simulink model "Moteurs_PLA"  (R2020b)
settings: Solver=FixedStepAuto  StartTime=0.0  StopTime=tsim+0.2  FixedStep=0.001  RelTol=1e-3
values from neighbouring files (symbols this model uses):
  X = C.Data(:,1,:)    [Initiliastion_PLA.m]
  x0 = -0.3929    [Simulation_PLA.m]
  x1 = -0.3929    [Simulation_PLA.m]
  xraten = a    (= 0)    [Simulation_PLA.m]
  xratep = 0    [Simulation_PLA.m]
  Y = C.Data(:,2,:)    [Initiliastion_PLA.m]
  y0 = -0.006639    [Simulation_PLA.m]
  y1 = -0.006639    [Simulation_PLA.m]
  yraten = b    (= 0)    [Simulation_PLA.m]
  yratep = 0    [Simulation_PLA.m]
  Z = C.Data(:,3,:)    [Initiliastion_PLA.m]
  z0 = 0.25    [Simulation_PLA.m]
  z1 = 0.25    [Simulation_PLA.m]
  zraten = c    (= 0)    [Simulation_PLA.m]
  zratep = 0    [Simulation_PLA.m]
undefined symbols (not defined in the file or in its folder): Levenberg, Marquardt, smiData
libraries: sm_lib x404, nesl_utility x24, robotcorelib x1, robotmaniplib x1
(part 1 of 7)
settings Model: Creator=alessandrini  LastModifiedBy=alessandrini
settings ExplorerConfigSet: InternalSimMechanicsExplorerSettings="<ExplorerConfiguration><canonicalview>default</canonicalview><AnimationSetting><BasePlaybackSpeed>1.0</BasePlaybackSpeed><PlaybackSpeedFactor>1.0</PlaybackSpeedFactor></AnimationSetting><TilePanel><TileInfo><Tiles Columns=\"1\" Count=\"1\" Rows=\"1\"><Column Weight=\"1\"/><Row Weight=\"1\"/><Tile Height=\"1\" Width=\"1\" X=\"0\" Y=\"0\"/></Tiles></TileInfo><SceneInfo><SceneViewer><BGColor><R>1</R><G>1</G><B>1</B></BGColor><Camera><DoPerspective>off</DoPerspective><Position><X>0.443375350255403866</X><Y>-0.57400040031573929</Y><Z>0.816945670282958059</Z></Position><Center><X>-0.133974918934221976</X><Y>0.00334986887388660781</Y><Z>0.239595401093332216</Z></Center><Up><X>-0.408248290463863073</X><Y>0.408248290463863073</Y><Z>0.816496580927726145</Z></Up><ViewLimDist>1</ViewLimDist><YLim>0.387829513549804716</YLim><XLim>0.326078018188476593</XLim></Camera></SceneViewer></SceneInfo></TilePanel><MechEditorPanel><Cameras/><GfxPanelCameraMap/><VideoCreator><PlaybackSpeedRatio>1.0</PlaybackSpeedRatio><FrameRate>30</FrameRate><VideoFormat>Motion JPEG AVI</VideoFormat><FrameSize>auto</FrameSize></VideoCreator></MechEditorPanel></ExplorerConfiguration>"

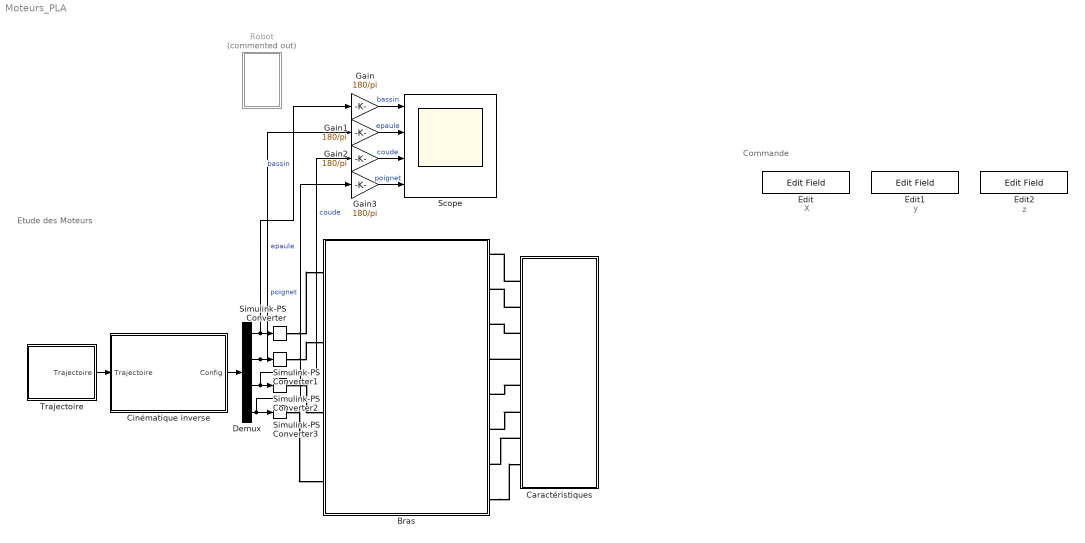
== system Moteurs_PLA ==
  note: Commande
  note: z
  note: y
  note: X
  note: Etude des Moteurs
  Bras : Subsystem
  Caractéristiques : Subsystem
  Cinématique inverse : Subsystem
  Demux : Demux
  Edit : EditField  LabelPosition=Hide  ShowInitialText=on  Alignment=Center
  Edit1 : EditField  LabelPosition=Hide  ShowInitialText=on  Alignment=Center
  Edit2 : EditField  LabelPosition=Hide  ShowInitialText=on  Alignment=Center
  Gain{,1..3} (4 alike) : Gain  Gain=180/pi
  Robot : Subsystem  Commented=on
  Scope : Scope  NumInputPorts=4
  Simulink-PS Converter{,1..3} (4 alike) : nesl_utility/Simulink-PS Converter  PhysicalDomain=network_engine_domain  SubClassName=ps_input  LeftPortType=input  RightPortType=output  PseudoPeriodic=off  Frequencies=[]  NoiseDistribution=none  NoiseParameters=[]  Unit=1  AffineConversion=off  FilteringAndDerivatives=filter  SimscapeFilterOrder=2  InputFilterTimeConstant=0.001  UdotUserProvided=0
  Trajectoire : Subsystem
  wires:
  Trajectoire/1(Trajectoire) -> Cinématique inverse/1(Trajectoire)
  Demux/4 -> Gain3/1, Simulink-PS Converter3/1  "poignet"
  Cinématique inverse/1(Config) -> Demux/1
  Gain/1 -> Scope/1  "bassin"
  Gain2/1 -> Scope/3  "coude"
  Demux/2 -> Gain1/1, Simulink-PS Converter1/1  "epaule"
  Gain1/1 -> Scope/2  "epaule"
  Demux/1 -> Gain/1, Simulink-PS Converter/1  "bassin"
  Demux/3 -> Gain2/1, Simulink-PS Converter2/1  "coude"
  Gain3/1 -> Scope/4  "poignet"
  connections:
  Caractéristiques/LConn1 -- Bras/RConn1
  Caractéristiques/LConn3 -- Bras/RConn3
  Caractéristiques/LConn5 -- Bras/RConn5
  Simulink-PS Converter1/RConn1 -- Bras/LConn2
  Caractéristiques/LConn4 -- Bras/RConn4
  Caractéristiques/LConn2 -- Bras/RConn2
  Caractéristiques/LConn6 -- Bras/RConn6
  Simulink-PS Converter/RConn1 -- Bras/LConn1
  Caractéristiques/LConn7 -- Bras/RConn7
  Simulink-PS Converter2/RConn1 -- Bras/LConn3
  Simulink-PS Converter3/RConn1 -- Bras/LConn4
  Bras/RConn8 -- Caractéristiques/LConn8

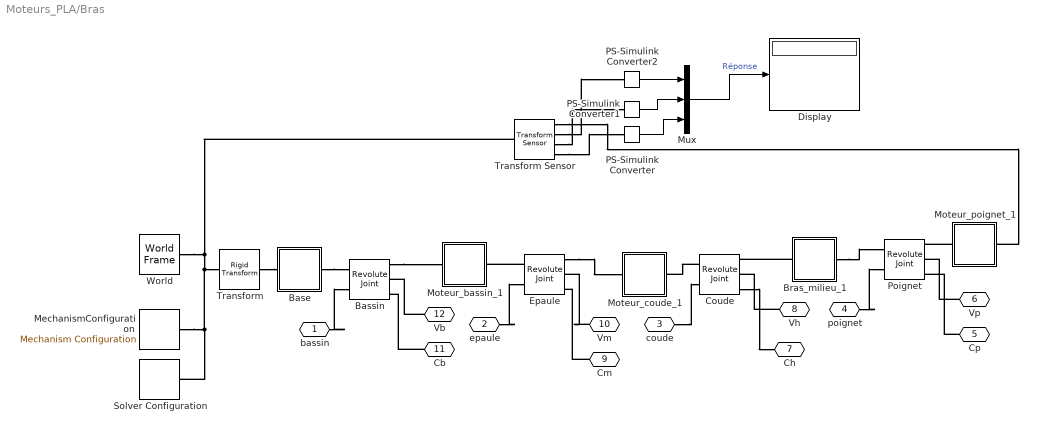
== system Moteurs_PLA/Bras ==
  Base : Subsystem
  Bassin : sm_lib/Joints/Revolute Joint  JointMode=Normal  SenseConstraintForce=off  SenseConstraintForceX=off  SenseConstraintForceY=off  SenseConstraintForceZ=off  SenseConstraintTorque=off  SenseConstraintTorqueX=off  SenseConstraintTorqueY=off  SenseConstraintTorqueZ=off  SenseTotalForce=off  SenseTotalForceX=off  SenseTotalForceY=off  SenseTotalForceZ=off  SenseTotalTorque=off  SenseTotalTorqueX=off  SenseTotalTorqueY=off  SenseTotalTorqueZ=off  CompositeWrenchDir=FollowerOnBase  CompositeWrenchFrame=BaseFrame  EquilibriumPosition=0  EquilibriumPositionUnits=deg  SpringStiffness=0  SpringStiffnessUnits=N*m/deg  DampingCoefficient=0  DampingCoefficientUnits=N*m/(deg/s)  TorqueActuationMode=ComputedTorque  MotionActuationMode=InputMotion  SensePosition=off  SenseVelocity=on  SenseAcceleration=off  SenseTorqueForce=on  SenseLowerLimitTorqueForce=off  SenseUpperLimitTorqueForce=off  LowerLimitSpecify=off  LowerLimitBound=-180  LowerLimitBoundUnits=deg  LowerLimitStiffness=1e4  LowerLimitStiffnessUnits=N*m/deg  LowerLimitDamping=10  LowerLimitDampingUnits=N*m/(deg/s)  LowerLimitTransitionRegionWidth=0.1  LowerLimitTransitionRegionWidthUnits=deg  UpperLimitSpecify=off  UpperLimitBound=180  UpperLimitBoundUnits=deg  UpperLimitStiffness=1e4  UpperLimitStiffnessUnits=N*m/deg  UpperLimitDamping=10  UpperLimitDampingUnits=N*m/(deg/s)  UpperLimitTransitionRegionWidth=0.1  UpperLimitTransitionRegionWidthUnits=deg  PositionTargetSpecify=on  PositionTargetPriority=Low  PositionTargetValue=smiData.RevoluteJoint(5).Rz.Pos  PositionTargetValueUnits=deg  VelocityTargetSpecify=off  VelocityTargetPriority=High  VelocityTargetValue=0  VelocityTargetValueUnits=deg/s
  Bras_milieu_1 : Subsystem
  Coude : sm_lib/Joints/Revolute Joint  JointMode=Normal  SenseConstraintForce=off  SenseConstraintForceX=off  SenseConstraintForceY=off  SenseConstraintForceZ=off  SenseConstraintTorque=off  SenseConstraintTorqueX=off  SenseConstraintTorqueY=off  SenseConstraintTorqueZ=off  SenseTotalForce=off  SenseTotalForceX=off  SenseTotalForceY=off  SenseTotalForceZ=off  SenseTotalTorque=off  SenseTotalTorqueX=off  SenseTotalTorqueY=off  SenseTotalTorqueZ=off  CompositeWrenchDir=FollowerOnBase  CompositeWrenchFrame=BaseFrame  EquilibriumPosition=0  EquilibriumPositionUnits=deg  SpringStiffness=0  SpringStiffnessUnits=N*m/deg  DampingCoefficient=0  DampingCoefficientUnits=N*m/(deg/s)  TorqueActuationMode=ComputedTorque  MotionActuationMode=InputMotion  SensePosition=off  SenseVelocity=on  SenseAcceleration=off  SenseTorqueForce=on  SenseLowerLimitTorqueForce=off  SenseUpperLimitTorqueForce=off  LowerLimitSpecify=on  LowerLimitBound=-110  LowerLimitBoundUnits=deg  LowerLimitStiffness=1e4  LowerLimitStiffnessUnits=N*m/deg  LowerLimitDamping=10  LowerLimitDampingUnits=N*m/(deg/s)  LowerLimitTransitionRegionWidth=0.1  LowerLimitTransitionRegionWidthUnits=deg  UpperLimitSpecify=on  UpperLimitBound=0  UpperLimitBoundUnits=deg  UpperLimitStiffness=1e4  UpperLimitStiffnessUnits=N*m/deg  UpperLimitDamping=10  UpperLimitDampingUnits=N*m/(deg/s)  UpperLimitTransitionRegionWidth=0.1  UpperLimitTransitionRegionWidthUnits=deg  PositionTargetSpecify=on  PositionTargetPriority=Low  PositionTargetValue=smiData.RevoluteJoint(2).Rz.Pos  PositionTargetValueUnits=deg  VelocityTargetSpecify=off  VelocityTargetPriority=High  VelocityTargetValue=0  VelocityTargetValueUnits=deg/s
  Display : Display
  Epaule : sm_lib/Joints/Revolute Joint  JointMode=Normal  SenseConstraintForce=off  SenseConstraintForceX=off  SenseConstraintForceY=off  SenseConstraintForceZ=off  SenseConstraintTorque=off  SenseConstraintTorqueX=off  SenseConstraintTorqueY=off  SenseConstraintTorqueZ=off  SenseTotalForce=off  SenseTotalForceX=off  SenseTotalForceY=off  SenseTotalForceZ=off  SenseTotalTorque=off  SenseTotalTorqueX=off  SenseTotalTorqueY=off  SenseTotalTorqueZ=off  CompositeWrenchDir=FollowerOnBase  CompositeWrenchFrame=BaseFrame  EquilibriumPosition=0  EquilibriumPositionUnits=deg  SpringStiffness=0  SpringStiffnessUnits=N*m/deg  DampingCoefficient=0  DampingCoefficientUnits=N*m/(deg/s)  TorqueActuationMode=ComputedTorque  MotionActuationMode=InputMotion  SensePosition=off  SenseVelocity=on  SenseAcceleration=off  SenseTorqueForce=on  SenseLowerLimitTorqueForce=off  SenseUpperLimitTorqueForce=off  LowerLimitSpecify=on  LowerLimitBound=0  LowerLimitBoundUnits=deg  LowerLimitStiffness=1e4  LowerLimitStiffnessUnits=N*m/deg  LowerLimitDamping=10  LowerLimitDampingUnits=N*m/(deg/s)  LowerLimitTransitionRegionWidth=0.1  LowerLimitTransitionRegionWidthUnits=deg  UpperLimitSpecify=on  UpperLimitBound=180  UpperLimitBoundUnits=deg  UpperLimitStiffness=1e4  UpperLimitStiffnessUnits=N*m/deg  UpperLimitDamping=10  UpperLimitDampingUnits=N*m/(deg/s)  UpperLimitTransitionRegionWidth=0.1  UpperLimitTransitionRegionWidthUnits=deg  PositionTargetSpecify=on  PositionTargetPriority=Low  PositionTargetValue=smiData.RevoluteJoint(4).Rz.Pos  PositionTargetValueUnits=deg  VelocityTargetSpecify=off  VelocityTargetPriority=High  VelocityTargetValue=0  VelocityTargetValueUnits=deg/s
  MechanismConfiguration : sm_lib/Utilities/Mechanism Configuration  UniformGravity=Constant  GravityVector=[0 0 -9.80665]  GravityVectorUnits=m/s^2  GravityUnits=m/s^2  LinearizationDelta=0.001  JointModeTransitionNonlinearIterations=2
  Moteur_bassin_1 : Subsystem
  Moteur_coude_1 : Subsystem
  Moteur_poignet_1 : Subsystem
  Mux : Mux  Inputs=3
  PS-Simulink Converter : nesl_utility/PS-Simulink Converter  PhysicalDomain=network_engine_domain  SubClassName=ps_output  LeftPortType=input  RightPortType=output  PseudoPeriodic=off  Frequencies=[]  Unit=inherit  AffineConversion=off
  PS-Simulink Converter1 : nesl_utility/PS-Simulink Converter  PhysicalDomain=network_engine_domain  SubClassName=ps_output  LeftPortType=input  RightPortType=output  PseudoPeriodic=off  Frequencies=[]  Unit=inherit  AffineConversion=off
  PS-Simulink Converter2 : nesl_utility/PS-Simulink Converter  PhysicalDomain=network_engine_domain  SubClassName=ps_output  LeftPortType=input  RightPortType=output  PseudoPeriodic=off  Frequencies=[]  Unit=inherit  AffineConversion=off
  Poignet : sm_lib/Joints/Revolute Joint  JointMode=Normal  SenseConstraintForce=off  SenseConstraintForceX=off  SenseConstraintForceY=off  SenseConstraintForceZ=off  SenseConstraintTorque=off  SenseConstraintTorqueX=off  SenseConstraintTorqueY=off  SenseConstraintTorqueZ=off  SenseTotalForce=off  SenseTotalForceX=off  SenseTotalForceY=off  SenseTotalForceZ=off  SenseTotalTorque=off  SenseTotalTorqueX=off  SenseTotalTorqueY=off  SenseTotalTorqueZ=off  CompositeWrenchDir=FollowerOnBase  CompositeWrenchFrame=BaseFrame  EquilibriumPosition=0  EquilibriumPositionUnits=deg  SpringStiffness=0  SpringStiffnessUnits=N*m/deg  DampingCoefficient=0  DampingCoefficientUnits=N*m/(deg/s)  TorqueActuationMode=ComputedTorque  MotionActuationMode=InputMotion  SensePosition=off  SenseVelocity=on  SenseAcceleration=off  SenseTorqueForce=on  SenseLowerLimitTorqueForce=off  SenseUpperLimitTorqueForce=off  LowerLimitSpecify=on  LowerLimitBound=30  LowerLimitBoundUnits=deg  LowerLimitStiffness=1e4  LowerLimitStiffnessUnits=N*m/deg  LowerLimitDamping=10  LowerLimitDampingUnits=N*m/(deg/s)  LowerLimitTransitionRegionWidth=0.1  LowerLimitTransitionRegionWidthUnits=deg  UpperLimitSpecify=on  UpperLimitBound=150  UpperLimitBoundUnits=deg  UpperLimitStiffness=1e4  UpperLimitStiffnessUnits=N*m/deg  UpperLimitDamping=10  UpperLimitDampingUnits=N*m/(deg/s)  UpperLimitTransitionRegionWidth=0.1  UpperLimitTransitionRegionWidthUnits=deg  PositionTargetSpecify=on  PositionTargetPriority=Low  PositionTargetValue=smiData.RevoluteJoint(3).Rz.Pos  PositionTargetValueUnits=deg  VelocityTargetSpecify=off  VelocityTargetPriority=High  VelocityTargetValue=0  VelocityTargetValueUnits=deg/s
  Solver Configuration : nesl_utility/Solver Configuration  PhysicalDomain=network_engine_domain  SubClassName=solver  LeftPortType=input  RightPortType=generic  Tones=[]  Harmonics=[]  SimulateNoise=off  Profile=off  UseLocalSampling=off  EnableSwitchedLinearOptims=on  FrequencyDomain=off  UseCCode=off  RelTol=0.001  AbsTol=1e-06  MinStep=1e-09  ToWorkspace=off  RevertToSquareIcSolve=off  NumHomotopyIterations=100  PhasorMode=off  PhasorModeNumHarmonics=1  DoDC=off  ResidualTolerance=1e-09  UseLocalSolver=off  LocalSolverChoice=NE_BACKWARD_EULER_ADVANCER  LocalSolverSampleTime=0.001  DoFixedCost=off  MaxNonlinIter=3  MaxModeIter=2  ComputeImpulses=off  ImpulseIterations=2  LinearAlgebra=auto  EquationFormulation=NE_TIME_EF  DelaysMemoryBudget=1024  AutomaticFiltering=on  FilteringTimeConstant=0.001  PartitionStorageMethod=AS_NEEDED  PartitionMemoryBudget=1024  PartitionMethod=ROBUST
  Transform : sm_lib/Frames and Transforms/Rigid Transform  TranslationMethod=Cartesian  TranslationStandardOffset=0  TranslationLengthUnit=m  TranslationStandardAxis=+Z  TranslationCartesianOffset=smiData.RigidTransform(93).translation  TranslationROffset=0  TranslationROffsetUnits=m  TranslationZOffset=0  TranslationZOffsetUnits=m  TranslationThetaOffset=0  TranslationThetaOffsetUnits=deg  RotationMethod=ArbitraryAxis  RotationAngleUnits=rad  RotationStandardAxis=+Z  RotationAngle=smiData.RigidTransform(93).angle  RotationArbitraryAxis=smiData.RigidTransform(93).axis  FollAlignAxisA=+X  BaseAlignAxisA=+Y  FollAlignAxisB=+Y  BaseAlignAxisB=+Z  RotationSequenceAxes=FollowerAxes  RotationSequence=XYX  RotationSequenceAngles=[0 0 0]  RotationSequenceAnglesUnits=deg  RotationMatrix=[1 0 0; 0 1 0; 0 0 1]
  Transform Sensor : sm_lib/Frames and Transforms/Transform Sensor  MeasurementFrame=World  SenseAngle=off  SenseAxis=off  SenseAngle1=off  SenseAngle2=off  SenseAngle3=off  SenseQ=off  SenseR=off  SenseOmegaX=off  SenseOmegaY=off  SenseOmegaZ=off  SenseOmega1=off  SenseOmega2=off  SenseOmega3=off  SenseQDot=off  SenseRDot=off  SenseAlphaX=off  SenseAlphaY=off  SenseAlphaZ=off  SenseAlpha1=off  SenseAlpha2=off  SenseAlpha3=off  SenseQDDot=off  SenseRDDot=off  SenseX=on  SenseY=on  SenseZ=on  SenseRad=off  SenseAzim=off  SenseDist=off  SenseInc=off  SenseXDot=off  SenseYDot=off  SenseZDot=off  SenseRadDot=off  SenseAzimDot=off  SenseDistDot=off  SenseIncDot=off  SenseXDDot=off  SenseYDDot=off  SenseZDDot=off  SenseRadDDot=off  SenseAzimDDot=off  SenseDistDDot=off  SenseIncDDot=off
  World : sm_lib/Frames and Transforms/World Frame
  bassin : PMIOPort  Side=Left
  epaule : PMIOPort  Port=2  Side=Left
  coude : PMIOPort  Port=3  Side=Left
  poignet : PMIOPort  Port=4  Side=Left
  Cp : PMIOPort  Port=5  Side=Right
  Vp : PMIOPort  Port=6  Side=Right
  Ch : PMIOPort  Port=7  Side=Right
  Vh : PMIOPort  Port=8  Side=Right
  Cm : PMIOPort  Port=9  Side=Right
  Vm : PMIOPort  Port=10  Side=Right
  Cb : PMIOPort  Port=11  Side=Right
  Vb : PMIOPort  Port=12  Side=Right
  wires:
  PS-Simulink Converter/1 -> Mux/3
  PS-Simulink Converter2/1 -> Mux/1
  PS-Simulink Converter1/1 -> Mux/2
  Mux/1 -> Display/1  "Réponse"
  connections:
  Solver Configuration/RConn1 -- Transform Sensor/LConn1 -- World/RConn1 -- Transform/LConn1 -- MechanismConfiguration/RConn1
  Base/RConn1 -- Bassin/LConn1
  Transform/RConn1 -- Base/LConn1
  Bras_milieu_1/RConn1 -- Poignet/LConn1
  Moteur_poignet_1/LConn1 -- Poignet/RConn1
  Epaule/LConn1 -- Moteur_bassin_1/RConn1
  Bassin/RConn1 -- Moteur_bassin_1/LConn1
  Bras_milieu_1/LConn1 -- Coude/RConn1
  Coude/LConn1 -- Moteur_coude_1/RConn1
  Epaule/RConn1 -- Moteur_coude_1/LConn1
  epaule/RConn1 -- Epaule/LConn2
  bassin/RConn1 -- Bassin/LConn2
  coude/RConn1 -- Coude/LConn2
  poignet/RConn1 -- Poignet/LConn2
  Vb/RConn1 -- Bassin/RConn2
  Cb/RConn1 -- Bassin/RConn3
  Vm/RConn1 -- Epaule/RConn2
  Cm/RConn1 -- Epaule/RConn3
  Vh/RConn1 -- Coude/RConn2
  Coude/RConn3 -- Ch/RConn1
  Vp/RConn1 -- Poignet/RConn2
  Cp/RConn1 -- Poignet/RConn3
  Transform Sensor/RConn4 -- PS-Simulink Converter/LConn1
  Transform Sensor/RConn3 -- PS-Simulink Converter1/LConn1
  Transform Sensor/RConn2 -- PS-Simulink Converter2/LConn1
  Transform Sensor/RConn1 -- Moteur_poignet_1/RConn1

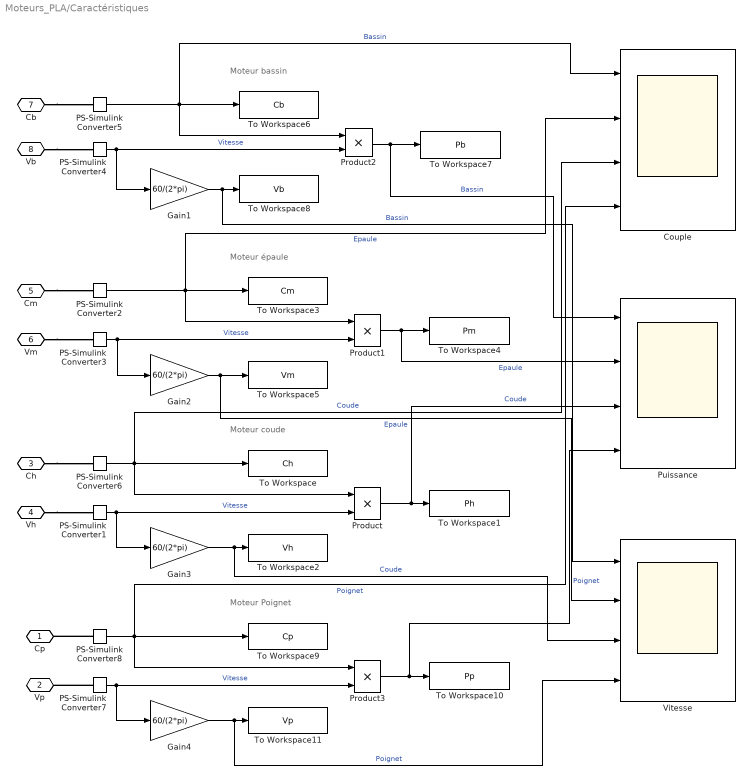
== system Moteurs_PLA/Caractéristiques ==
  note: Moteur coude
  note: Moteur épaule
  note: Moteur bassin
  note: Moteur Poignet
  Couple : Scope  NumInputPorts=4
  Gain{1..4} (4 alike) : Gain  Gain=60/(2*pi)
  PS-Simulink Converter{1..8} (8 alike) : nesl_utility/PS-Simulink Converter  PhysicalDomain=network_engine_domain  SubClassName=ps_output  LeftPortType=input  RightPortType=output  PseudoPeriodic=off  Frequencies=[]  Unit=inherit  AffineConversion=off
  Product{,1..3} (4 alike) : Product
  Puissance : Scope  NumInputPorts=4
  To Workspace : ToWorkspace  VariableName=Ch  SaveFormat=Timeseries  SampleTime=-1
  To Workspace1 : ToWorkspace  VariableName=Ph  SaveFormat=Timeseries  SampleTime=-1
  To Workspace10 : ToWorkspace  VariableName=Pp  SaveFormat=Timeseries  SampleTime=-1
  To Workspace11 : ToWorkspace  VariableName=Vp  SaveFormat=Timeseries  SampleTime=-1
  To Workspace2 : ToWorkspace  VariableName=Vh  SaveFormat=Timeseries  SampleTime=-1
  To Workspace3 : ToWorkspace  VariableName=Cm  SaveFormat=Timeseries  SampleTime=-1
  To Workspace4 : ToWorkspace  VariableName=Pm  SaveFormat=Timeseries  SampleTime=-1
  To Workspace5 : ToWorkspace  VariableName=Vm  SaveFormat=Timeseries  SampleTime=-1
  To Workspace6 : ToWorkspace  VariableName=Cb  SaveFormat=Timeseries  SampleTime=-1
  To Workspace7 : ToWorkspace  VariableName=Pb  SaveFormat=Timeseries  SampleTime=-1
  To Workspace8 : ToWorkspace  VariableName=Vb  SaveFormat=Timeseries  SampleTime=-1
  To Workspace9 : ToWorkspace  VariableName=Cp  SaveFormat=Timeseries  SampleTime=-1
  Vitesse : Scope  NumInputPorts=4
  Cp : PMIOPort  Side=Left
  Vp : PMIOPort  Port=2  Side=Left
  Ch : PMIOPort  Port=3  Side=Left
  Vh : PMIOPort  Port=4  Side=Left
  Cm : PMIOPort  Port=5  Side=Left
  Vm : PMIOPort  Port=6  Side=Left
  Cb : PMIOPort  Port=7  Side=Left
  Vb : PMIOPort  Port=8  Side=Left
  wires:
  Gain4/1 -> Vitesse/4, To Workspace11/1  "Poignet"
  Product3/1 -> Puissance/4, To Workspace10/1  "Poignet"
  Gain1/1 -> Vitesse/1, To Workspace8/1  "Bassin"
  PS-Simulink Converter2/1 -> Couple/2, To Workspace3/1, Product1/1  "Epaule"
  PS-Simulink Converter3/1 -> Gain2/1, Product1/2  "Vitesse"
  Product2/1 -> Puissance/1, To Workspace7/1  "Bassin"
  PS-Simulink Converter6/1 -> Couple/3, Product/1, To Workspace/1  "Coude"
  PS-Simulink Converter7/1 -> Gain4/1, Product3/2  "Vitesse"
  Product/1 -> Puissance/3, To Workspace1/1  "Coude"
  Gain3/1 -> Vitesse/3, To Workspace2/1  "Coude"
  PS-Simulink Converter1/1 -> Gain3/1, Product/2  "Vitesse"
  PS-Simulink Converter8/1 -> Couple/4, Product3/1, To Workspace9/1  "Poignet"
  Gain2/1 -> Vitesse/2, To Workspace5/1  "Epaule"
  Product1/1 -> Puissance/2, To Workspace4/1  "Epaule"
  PS-Simulink Converter4/1 -> Gain1/1, Product2/2  "Vitesse"
  PS-Simulink Converter5/1 -> Couple/1, To Workspace6/1, Product2/1  "Bassin"
  connections:
  PS-Simulink Converter7/LConn1 -- Vp/RConn1
  Vm/RConn1 -- PS-Simulink Converter3/LConn1
  PS-Simulink Converter8/LConn1 -- Cp/RConn1
  Vh/RConn1 -- PS-Simulink Converter1/LConn1
  Vb/RConn1 -- PS-Simulink Converter4/LConn1
  Cm/RConn1 -- PS-Simulink Converter2/LConn1
  Ch/RConn1 -- PS-Simulink Converter6/LConn1
  Cb/RConn1 -- PS-Simulink Converter5/LConn1

== system Moteurs_PLA/Cinématique inverse ==
  Trajectoire : Inport
  Constant1 : Constant  Value=[0 0 0 1 1 1]  VectorParams1D=off
  Coordinate Transformation Conversion1 : robotcorelib/Coordinate Transformation Conversion  InputRepresentation=Translation Vector  InputEulerSequence=ZYX  ShowTrVecInputPort=on  OutputRepresentation=Homogeneous Transformation  OutputEulerSequence=ZYX  ShowTrVecOutputPort=on  SimulateUsing=Interpreted execution
  Delay : Delay  DelayLength=1  InitialCondition=([0 -10 0 90]*pi/180)'
  Inverse Kinematics : robotmaniplib/Inverse Kinematics  RigidBodyTree=robot  EndEffector=Body5  ShowInfo=on  SolverName=Levenberg-Marquardt  EnforceJointLimits=on  MaxIterations=1500  MaxTime=10  GradientTolerance=1e-7  SolutionTolerance=1e-6  StepTolerance=1e-14  ErrorChangeTolerance=1e-12  UseErrorDamping=on  DampingBias=0.0025  SimulateUsing=Interpreted execution
  Terminator : Terminator
  Config : Outport
  wires:
  Coordinate Transformation Conversion1/1 -> Inverse Kinematics/1
  Delay/1 -> Inverse Kinematics/3
  Constant1/1 -> Inverse Kinematics/2
  Trajectoire/1 -> Coordinate Transformation Conversion1/1
  Inverse Kinematics/2 -> Terminator/1
  Inverse Kinematics/1 -> Config/1, Delay/1

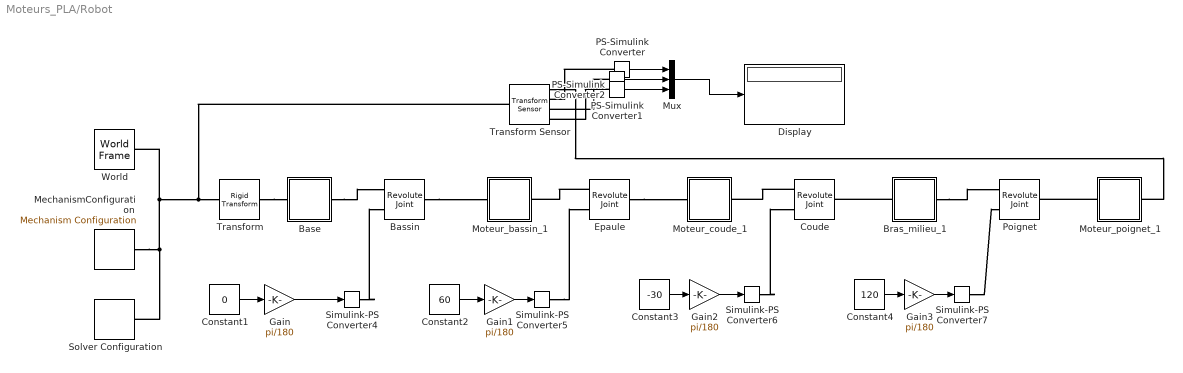
== system Moteurs_PLA/Robot ==
  Base : Subsystem
  Bassin : sm_lib/Joints/Revolute Joint  JointMode=Normal  SenseConstraintForce=off  SenseConstraintForceX=off  SenseConstraintForceY=off  SenseConstraintForceZ=off  SenseConstraintTorque=off  SenseConstraintTorqueX=off  SenseConstraintTorqueY=off  SenseConstraintTorqueZ=off  SenseTotalForce=off  SenseTotalForceX=off  SenseTotalForceY=off  SenseTotalForceZ=off  SenseTotalTorque=off  SenseTotalTorqueX=off  SenseTotalTorqueY=off  SenseTotalTorqueZ=off  CompositeWrenchDir=FollowerOnBase  CompositeWrenchFrame=BaseFrame  EquilibriumPosition=0  EquilibriumPositionUnits=deg  SpringStiffness=0  SpringStiffnessUnits=N*m/deg  DampingCoefficient=0  DampingCoefficientUnits=N*m/(deg/s)  TorqueActuationMode=ComputedTorque  MotionActuationMode=InputMotion  SensePosition=off  SenseVelocity=off  SenseAcceleration=off  SenseTorqueForce=off  SenseLowerLimitTorqueForce=off  SenseUpperLimitTorqueForce=off  LowerLimitSpecify=off  LowerLimitBound=0  LowerLimitBoundUnits=deg  LowerLimitStiffness=1e4  LowerLimitStiffnessUnits=N*m/deg  LowerLimitDamping=10  LowerLimitDampingUnits=N*m/(deg/s)  LowerLimitTransitionRegionWidth=0.1  LowerLimitTransitionRegionWidthUnits=deg  UpperLimitSpecify=off  UpperLimitBound=360  UpperLimitBoundUnits=deg  UpperLimitStiffness=1e4  UpperLimitStiffnessUnits=N*m/deg  UpperLimitDamping=10  UpperLimitDampingUnits=N*m/(deg/s)  UpperLimitTransitionRegionWidth=0.1  UpperLimitTransitionRegionWidthUnits=deg  PositionTargetSpecify=on  PositionTargetPriority=Low  PositionTargetValue=smiData.RevoluteJoint(5).Rz.Pos  PositionTargetValueUnits=deg  VelocityTargetSpecify=off  VelocityTargetPriority=High  VelocityTargetValue=0  VelocityTargetValueUnits=deg/s
  Bras_milieu_1 : Subsystem
  Constant1 : Constant  Value=0
  Constant2 : Constant  Value=60
  Constant3 : Constant  Value=-30
  Constant4 : Constant  Value=120
  Coude : sm_lib/Joints/Revolute Joint  JointMode=Normal  SenseConstraintForce=off  SenseConstraintForceX=off  SenseConstraintForceY=off  SenseConstraintForceZ=off  SenseConstraintTorque=off  SenseConstraintTorqueX=off  SenseConstraintTorqueY=off  SenseConstraintTorqueZ=off  SenseTotalForce=off  SenseTotalForceX=off  SenseTotalForceY=off  SenseTotalForceZ=off  SenseTotalTorque=off  SenseTotalTorqueX=off  SenseTotalTorqueY=off  SenseTotalTorqueZ=off  CompositeWrenchDir=FollowerOnBase  CompositeWrenchFrame=BaseFrame  EquilibriumPosition=0  EquilibriumPositionUnits=deg  SpringStiffness=0  SpringStiffnessUnits=N*m/deg  DampingCoefficient=0  DampingCoefficientUnits=N*m/(deg/s)  TorqueActuationMode=ComputedTorque  MotionActuationMode=InputMotion  SensePosition=off  SenseVelocity=off  SenseAcceleration=off  SenseTorqueForce=off  SenseLowerLimitTorqueForce=off  SenseUpperLimitTorqueForce=off  LowerLimitSpecify=on  LowerLimitBound=-110  LowerLimitBoundUnits=deg  LowerLimitStiffness=1e4  LowerLimitStiffnessUnits=N*m/deg  LowerLimitDamping=10  LowerLimitDampingUnits=N*m/(deg/s)  LowerLimitTransitionRegionWidth=0.1  LowerLimitTransitionRegionWidthUnits=deg  UpperLimitSpecify=on  UpperLimitBound=0  UpperLimitBoundUnits=deg  UpperLimitStiffness=1e4  UpperLimitStiffnessUnits=N*m/deg  UpperLimitDamping=10  UpperLimitDampingUnits=N*m/(deg/s)  UpperLimitTransitionRegionWidth=0.1  UpperLimitTransitionRegionWidthUnits=deg  PositionTargetSpecify=on  PositionTargetPriority=Low  PositionTargetValue=smiData.RevoluteJoint(2).Rz.Pos  PositionTargetValueUnits=deg  VelocityTargetSpecify=off  VelocityTargetPriority=High  VelocityTargetValue=0  VelocityTargetValueUnits=deg/s
  Display : Display
  Epaule : sm_lib/Joints/Revolute Joint  JointMode=Normal  SenseConstraintForce=off  SenseConstraintForceX=off  SenseConstraintForceY=off  SenseConstraintForceZ=off  SenseConstraintTorque=off  SenseConstraintTorqueX=off  SenseConstraintTorqueY=off  SenseConstraintTorqueZ=off  SenseTotalForce=off  SenseTotalForceX=off  SenseTotalForceY=off  SenseTotalForceZ=off  SenseTotalTorque=off  SenseTotalTorqueX=off  SenseTotalTorqueY=off  SenseTotalTorqueZ=off  CompositeWrenchDir=FollowerOnBase  CompositeWrenchFrame=BaseFrame  EquilibriumPosition=0  EquilibriumPositionUnits=deg  SpringStiffness=0  SpringStiffnessUnits=N*m/deg  DampingCoefficient=0  DampingCoefficientUnits=N*m/(deg/s)  TorqueActuationMode=ComputedTorque  MotionActuationMode=InputMotion  SensePosition=off  SenseVelocity=off  SenseAcceleration=off  SenseTorqueForce=off  SenseLowerLimitTorqueForce=off  SenseUpperLimitTorqueForce=off  LowerLimitSpecify=on  LowerLimitBound=60  LowerLimitBoundUnits=deg  LowerLimitStiffness=1e4  LowerLimitStiffnessUnits=N*m/deg  LowerLimitDamping=10  LowerLimitDampingUnits=N*m/(deg/s)  LowerLimitTransitionRegionWidth=0.1  LowerLimitTransitionRegionWidthUnits=deg  UpperLimitSpecify=on  UpperLimitBound=180  UpperLimitBoundUnits=deg  UpperLimitStiffness=1e4  UpperLimitStiffnessUnits=N*m/deg  UpperLimitDamping=10  UpperLimitDampingUnits=N*m/(deg/s)  UpperLimitTransitionRegionWidth=0.1  UpperLimitTransitionRegionWidthUnits=deg  PositionTargetSpecify=on  PositionTargetPriority=Low  PositionTargetValue=smiData.RevoluteJoint(4).Rz.Pos  PositionTargetValueUnits=deg  VelocityTargetSpecify=off  VelocityTargetPriority=High  VelocityTargetValue=0  VelocityTargetValueUnits=deg/s
  Gain{,1..3} (4 alike) : Gain  Gain=pi/180
  MechanismConfiguration : sm_lib/Utilities/Mechanism Configuration  UniformGravity=Constant  GravityVector=[0 0 -9.80665]  GravityVectorUnits=m/s^2  GravityUnits=m/s^2  LinearizationDelta=0.001  JointModeTransitionNonlinearIterations=2
  Moteur_bassin_1 : Subsystem
  Moteur_coude_1 : Subsystem
  Moteur_poignet_1 : Subsystem
  Mux : Mux  Inputs=3
  PS-Simulink Converter : nesl_utility/PS-Simulink Converter  PhysicalDomain=network_engine_domain  SubClassName=ps_output  LeftPortType=input  RightPortType=output  PseudoPeriodic=off  Frequencies=[]  Unit=inherit  AffineConversion=off
  PS-Simulink Converter1 : nesl_utility/PS-Simulink Converter  PhysicalDomain=network_engine_domain  SubClassName=ps_output  LeftPortType=input  RightPortType=output  PseudoPeriodic=off  Frequencies=[]  Unit=inherit  AffineConversion=off
  PS-Simulink Converter2 : nesl_utility/PS-Simulink Converter  PhysicalDomain=network_engine_domain  SubClassName=ps_output  LeftPortType=input  RightPortType=output  PseudoPeriodic=off  Frequencies=[]  Unit=inherit  AffineConversion=off
  Poignet : sm_lib/Joints/Revolute Joint  JointMode=Normal  SenseConstraintForce=off  SenseConstraintForceX=off  SenseConstraintForceY=off  SenseConstraintForceZ=off  SenseConstraintTorque=off  SenseConstraintTorqueX=off  SenseConstraintTorqueY=off  SenseConstraintTorqueZ=off  SenseTotalForce=off  SenseTotalForceX=off  SenseTotalForceY=off  SenseTotalForceZ=off  SenseTotalTorque=off  SenseTotalTorqueX=off  SenseTotalTorqueY=off  SenseTotalTorqueZ=off  CompositeWrenchDir=FollowerOnBase  CompositeWrenchFrame=BaseFrame  EquilibriumPosition=0  EquilibriumPositionUnits=deg  SpringStiffness=0  SpringStiffnessUnits=N*m/deg  DampingCoefficient=0  DampingCoefficientUnits=N*m/(deg/s)  TorqueActuationMode=ComputedTorque  MotionActuationMode=InputMotion  SensePosition=off  SenseVelocity=off  SenseAcceleration=off  SenseTorqueForce=off  SenseLowerLimitTorqueForce=off  SenseUpperLimitTorqueForce=off  LowerLimitSpecify=on  LowerLimitBound=30  LowerLimitBoundUnits=deg  LowerLimitStiffness=1e4  LowerLimitStiffnessUnits=N*m/deg  LowerLimitDamping=10  LowerLimitDampingUnits=N*m/(deg/s)  LowerLimitTransitionRegionWidth=0.1  LowerLimitTransitionRegionWidthUnits=deg  UpperLimitSpecify=on  UpperLimitBound=150  UpperLimitBoundUnits=deg  UpperLimitStiffness=1e4  UpperLimitStiffnessUnits=N*m/deg  UpperLimitDamping=10  UpperLimitDampingUnits=N*m/(deg/s)  UpperLimitTransitionRegionWidth=0.1  UpperLimitTransitionRegionWidthUnits=deg  PositionTargetSpecify=on  PositionTargetPriority=Low  PositionTargetValue=smiData.RevoluteJoint(3).Rz.Pos  PositionTargetValueUnits=deg  VelocityTargetSpecify=off  VelocityTargetPriority=High  VelocityTargetValue=0  VelocityTargetValueUnits=deg/s
  Simulink-PS Converter{4..7} (4 alike) : nesl_utility/Simulink-PS Converter  PhysicalDomain=network_engine_domain  SubClassName=ps_input  LeftPortType=input  RightPortType=output  PseudoPeriodic=off  Frequencies=[]  NoiseDistribution=none  NoiseParameters=[]  Unit=1  AffineConversion=off  FilteringAndDerivatives=provide  SimscapeFilterOrder=1  InputFilterTimeConstant=0.001  UdotUserProvided=0
  Solver Configuration : nesl_utility/Solver Configuration  PhysicalDomain=network_engine_domain  SubClassName=solver  LeftPortType=input  RightPortType=generic  Tones=[]  Harmonics=[]  SimulateNoise=off  Profile=off  UseLocalSampling=off  EnableSwitchedLinearOptims=on  FrequencyDomain=off  UseCCode=off  RelTol=0.001  AbsTol=1e-06  MinStep=1e-09  ToWorkspace=off  RevertToSquareIcSolve=off  NumHomotopyIterations=100  PhasorMode=off  PhasorModeNumHarmonics=1  DoDC=off  ResidualTolerance=1e-09  UseLocalSolver=off  LocalSolverChoice=NE_BACKWARD_EULER_ADVANCER  LocalSolverSampleTime=0.001  DoFixedCost=off  MaxNonlinIter=3  MaxModeIter=2  ComputeImpulses=off  ImpulseIterations=2  LinearAlgebra=auto  EquationFormulation=NE_TIME_EF  DelaysMemoryBudget=1024  AutomaticFiltering=on  FilteringTimeConstant=0.001  PartitionStorageMethod=AS_NEEDED  PartitionMemoryBudget=1024  PartitionMethod=ROBUST
  Transform : sm_lib/Frames and Transforms/Rigid Transform  TranslationMethod=Cartesian  TranslationStandardOffset=0  TranslationLengthUnit=m  TranslationStandardAxis=+Z  TranslationCartesianOffset=smiData.RigidTransform(93).translation  TranslationROffset=0  TranslationROffsetUnits=m  TranslationZOffset=0  TranslationZOffsetUnits=m  TranslationThetaOffset=0  TranslationThetaOffsetUnits=deg  RotationMethod=ArbitraryAxis  RotationAngleUnits=rad  RotationStandardAxis=+Z  RotationAngle=smiData.RigidTransform(93).angle  RotationArbitraryAxis=smiData.RigidTransform(93).axis  FollAlignAxisA=+X  BaseAlignAxisA=+Y  FollAlignAxisB=+Y  BaseAlignAxisB=+Z  RotationSequenceAxes=FollowerAxes  RotationSequence=XYX  RotationSequenceAngles=[0 0 0]  RotationSequenceAnglesUnits=deg  RotationMatrix=[1 0 0; 0 1 0; 0 0 1]
  Transform Sensor : sm_lib/Frames and Transforms/Transform Sensor  MeasurementFrame=World  SenseAngle=off  SenseAxis=off  SenseAngle1=off  SenseAngle2=off  SenseAngle3=off  SenseQ=off  SenseR=off  SenseOmegaX=off  SenseOmegaY=off  SenseOmegaZ=off  SenseOmega1=off  SenseOmega2=off  SenseOmega3=off  SenseQDot=off  SenseRDot=off  SenseAlphaX=off  SenseAlphaY=off  SenseAlphaZ=off  SenseAlpha1=off  SenseAlpha2=off  SenseAlpha3=off  SenseQDDot=off  SenseRDDot=off  SenseX=on  SenseY=on  SenseZ=on  SenseRad=off  SenseAzim=off  SenseDist=off  SenseInc=off  SenseXDot=off  SenseYDot=off  SenseZDot=off  SenseRadDot=off  SenseAzimDot=off  SenseDistDot=off  SenseIncDot=off  SenseXDDot=off  SenseYDDot=off  SenseZDDot=off  SenseRadDDot=off  SenseAzimDDot=off  SenseDistDDot=off  SenseIncDDot=off
  World : sm_lib/Frames and Transforms/World Frame
  wires:
  PS-Simulink Converter/1 -> Mux/1
  Constant4/1 -> Gain3/1
  Mux/1 -> Display/1
  Constant2/1 -> Gain1/1
  Gain1/1 -> Simulink-PS Converter5/1
  Gain2/1 -> Simulink-PS Converter6/1
  PS-Simulink Converter1/1 -> Mux/2
  Gain/1 -> Simulink-PS Converter4/1
  PS-Simulink Converter2/1 -> Mux/3
  Constant1/1 -> Gain/1
  Constant3/1 -> Gain2/1
  Gain3/1 -> Simulink-PS Converter7/1
  connections:
  Coude/LConn1 -- Moteur_coude_1/RConn1
  Simulink-PS Converter7/RConn1 -- Poignet/LConn2
  Transform/RConn1 -- Base/LConn1
  Simulink-PS Converter6/RConn1 -- Coude/LConn2
  Bassin/RConn1 -- Moteur_bassin_1/LConn1
  Moteur_poignet_1/LConn1 -- Poignet/RConn1
  Epaule/RConn1 -- Moteur_coude_1/LConn1
  Simulink-PS Converter4/RConn1 -- Bassin/LConn2
  PS-Simulink Converter1/LConn1 -- Transform Sensor/RConn3
  World/RConn1 -- Transform Sensor/LConn1 -- Transform/LConn1 -- MechanismConfiguration/RConn1 -- Solver Configuration/RConn1
  Base/RConn1 -- Bassin/LConn1
  Epaule/LConn1 -- Moteur_bassin_1/RConn1
  PS-Simulink Converter2/LConn1 -- Transform Sensor/RConn4
  Bras_milieu_1/LConn1 -- Coude/RConn1
  Bras_milieu_1/RConn1 -- Poignet/LConn1
  PS-Simulink Converter/LConn1 -- Transform Sensor/RConn2
  Transform Sensor/RConn1 -- Moteur_poignet_1/RConn1
  Simulink-PS Converter5/RConn1 -- Epaule/LConn2

== system Moteurs_PLA/Trajectoire ==
  Mux : Mux  Inputs=3
  Rate Limiter : RateLimiter  RisingSlewLimit=xratep  FallingSlewLimit=xraten  SampleTimeMode=inherited  InitialCondition=x0  LinearizeAsGain=off
  Rate Limiter1 : RateLimiter  RisingSlewLimit=yratep  FallingSlewLimit=yraten  SampleTimeMode=inherited  InitialCondition=y0  LinearizeAsGain=off
  Rate Limiter2 : RateLimiter  RisingSlewLimit=zratep  FallingSlewLimit=zraten  SampleTimeMode=inherited  InitialCondition=z0  LinearizeAsGain=off
  Step : Step  Time=0.323076923076923  Before=x0  After=x1  SampleTime=0.001
  Step1 : Step  Time=31.00328947368421  Before=y0  After=y1  SampleTime=0.001
  Step2 : Step  Time=0.1  Before=z0  After=z1  SampleTime=0.001
  To Workspace12 : ToWorkspace  VariableName=courbe  SaveFormat=Timeseries  SampleTime=-1
  Trajectoire : Outport
  wires:
  Rate Limiter/1 -> Mux/1
  Step1/1 -> Rate Limiter1/1
  Step/1 -> Rate Limiter/1
  Rate Limiter1/1 -> Mux/2
  Mux/1 -> Trajectoire/1, To Workspace12/1  "Consigne"
  Rate Limiter2/1 -> Mux/3
  Step2/1 -> Rate Limiter2/1

== system Moteurs_PLA/Bras/Base ==
  Base_1_RIGID : Subsystem
  Couvercle_1_RIGID : Subsystem
  Joints_1_RIGID : Subsystem
  F : PMIOPort  Side=Right
  F2 : PMIOPort  Port=2  Side=Left
  connections:
  Base_1_RIGID/LConn1 -- Joints_1_RIGID/LConn1
  Base_1_RIGID/LConn3 -- Couvercle_1_RIGID/LConn1
  Joints_1_RIGID/RConn1 -- F/RConn1
  F2/RConn1 -- Base_1_RIGID/LConn2

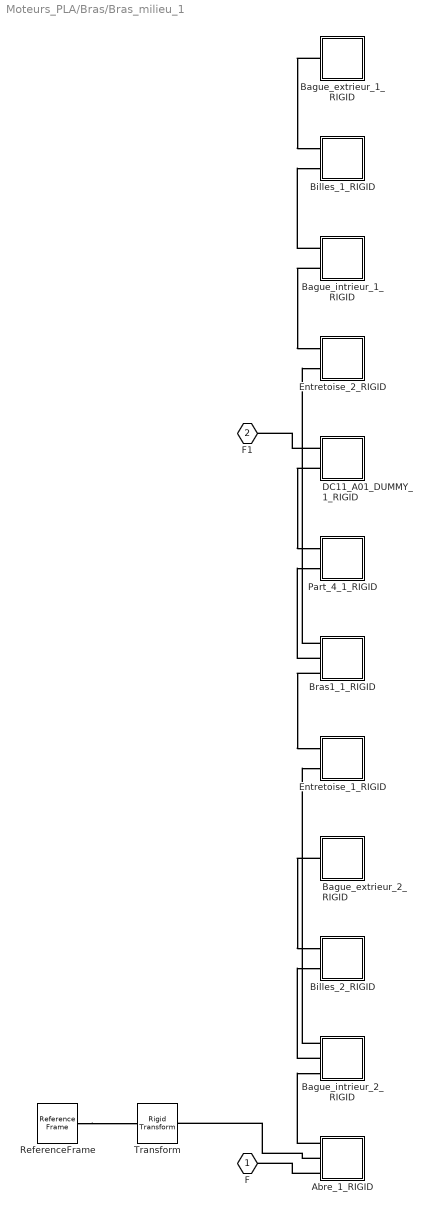
== system Moteurs_PLA/Bras/Bras_milieu_1 ==
  Abre_1_RIGID : Subsystem
  Bague_extrieur_1_RIGID : Subsystem
  Bague_extrieur_2_RIGID : Subsystem
  Bague_intrieur_1_RIGID : Subsystem
  Bague_intrieur_2_RIGID : Subsystem
  Billes_1_RIGID : Subsystem
  Billes_2_RIGID : Subsystem
  Bras1_1_RIGID : Subsystem
  DC11_A01_DUMMY_1_RIGID : Subsystem
  Entretoise_1_RIGID : Subsystem
  Entretoise_2_RIGID : Subsystem
  Part_4_1_RIGID : Subsystem
  ReferenceFrame : sm_lib/Frames and Transforms/Reference Frame
  Transform : sm_lib/Frames and Transforms/Rigid Transform  TranslationMethod=Cartesian  TranslationStandardOffset=0  TranslationLengthUnit=m  TranslationStandardAxis=+Z  TranslationCartesianOffset=smiData.RigidTransform(95).translation  TranslationROffset=0  TranslationROffsetUnits=m  TranslationZOffset=0  TranslationZOffsetUnits=m  TranslationThetaOffset=0  TranslationThetaOffsetUnits=deg  RotationMethod=ArbitraryAxis  RotationAngleUnits=rad  RotationStandardAxis=+Z  RotationAngle=smiData.RigidTransform(95).angle  RotationArbitraryAxis=smiData.RigidTransform(95).axis  FollAlignAxisA=+X  BaseAlignAxisA=+Y  FollAlignAxisB=+Y  BaseAlignAxisB=+Z  RotationSequenceAxes=FollowerAxes  RotationSequence=XYX  RotationSequenceAngles=[0 0 0]  RotationSequenceAnglesUnits=deg  RotationMatrix=[1 0 0; 0 1 0; 0 0 1]
  F : PMIOPort  Side=Left
  F1 : PMIOPort  Port=2  Side=Right
  connections:
  Abre_1_RIGID/LConn1 -- Bague_intrieur_2_RIGID/LConn3
  Bras1_1_RIGID/LConn2 -- Part_4_1_RIGID/LConn2
  Bague_intrieur_1_RIGID/LConn2 -- Entretoise_2_RIGID/LConn1
  Abre_1_RIGID/LConn3 -- F/RConn1
  DC11_A01_DUMMY_1_RIGID/LConn1 -- F1/RConn1
  Abre_1_RIGID/LConn2 -- Transform/RConn1
  ReferenceFrame/RConn1 -- Transform/LConn1
  DC11_A01_DUMMY_1_RIGID/LConn2 -- Part_4_1_RIGID/LConn1
  Bague_extrieur_2_RIGID/LConn1 -- Billes_2_RIGID/LConn1
  Bague_intrieur_2_RIGID/LConn2 -- Billes_2_RIGID/LConn2
  Bras1_1_RIGID/LConn3 -- Entretoise_1_RIGID/LConn1
  Bras1_1_RIGID/LConn1 -- Entretoise_2_RIGID/LConn2
  Bague_extrieur_1_RIGID/LConn1 -- Billes_1_RIGID/LConn1
  Bague_intrieur_1_RIGID/LConn1 -- Billes_1_RIGID/LConn2
  Bague_intrieur_2_RIGID/LConn1 -- Entretoise_1_RIGID/LConn2

== system Moteurs_PLA/Bras/Moteur_bassin_1 ==
  Bras0_1_RIGID : Subsystem
  Bras0_2_RIGID : Subsystem
  Fixation_moteur_1_RIGID : Subsystem
  Moteur_1_RIGID : Subsystem
  Mt_1_RIGID : Subsystem
  ReferenceFrame : sm_lib/Frames and Transforms/Reference Frame
  F1 : PMIOPort  Side=Left
  F : PMIOPort  Port=2  Side=Right
  connections:
  Bras0_1_RIGID/LConn2 -- Mt_1_RIGID/LConn1
  Bras0_1_RIGID/LConn1 -- Fixation_moteur_1_RIGID/LConn2
  Bras0_2_RIGID/LConn1 -- Mt_1_RIGID/LConn3
  Fixation_moteur_1_RIGID/LConn1 -- Moteur_1_RIGID/LConn2
  Moteur_1_RIGID/LConn1 -- F/RConn1
  Mt_1_RIGID/LConn2 -- F1/RConn1

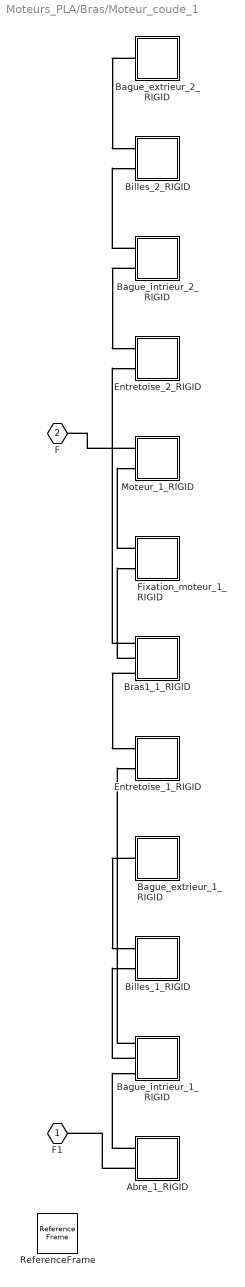
== system Moteurs_PLA/Bras/Moteur_coude_1 ==
  Abre_1_RIGID : Subsystem
  Bague_extrieur_1_RIGID : Subsystem
  Bague_extrieur_2_RIGID : Subsystem
  Bague_intrieur_1_RIGID : Subsystem
  Bague_intrieur_2_RIGID : Subsystem
  Billes_1_RIGID : Subsystem
  Billes_2_RIGID : Subsystem
  Bras1_1_RIGID : Subsystem
  Entretoise_1_RIGID : Subsystem
  Entretoise_2_RIGID : Subsystem
  Fixation_moteur_1_RIGID : Subsystem
  Moteur_1_RIGID : Subsystem
  ReferenceFrame : sm_lib/Frames and Transforms/Reference Frame
  F1 : PMIOPort  Side=Left
  F : PMIOPort  Port=2  Side=Right
  connections:
  Bras1_1_RIGID/LConn1 -- Entretoise_2_RIGID/LConn2
  Bras1_1_RIGID/LConn3 -- Entretoise_1_RIGID/LConn1
  Bague_intrieur_2_RIGID/LConn1 -- Billes_2_RIGID/LConn2
  Moteur_1_RIGID/LConn1 -- F/RConn1
  Abre_1_RIGID/LConn2 -- F1/RConn1
  Bras1_1_RIGID/LConn2 -- Fixation_moteur_1_RIGID/LConn2
  Fixation_moteur_1_RIGID/LConn1 -- Moteur_1_RIGID/LConn2
  Bague_extrieur_1_RIGID/LConn1 -- Billes_1_RIGID/LConn1
  Bague_intrieur_1_RIGID/LConn2 -- Billes_1_RIGID/LConn2
  Abre_1_RIGID/LConn1 -- Bague_intrieur_1_RIGID/LConn3
  Bague_extrieur_2_RIGID/LConn1 -- Billes_2_RIGID/LConn1
  Bague_intrieur_2_RIGID/LConn2 -- Entretoise_2_RIGID/LConn1
  Bague_intrieur_1_RIGID/LConn1 -- Entretoise_1_RIGID/LConn2

== system Moteurs_PLA/Bras/Moteur_poignet_1 ==
  Arbre_Poignet_1_RIGID : Subsystem
  Assemblage_Parfait_1 : Subsystem
  Goupille_1_RIGID : Subsystem
  Part_2_1_RIGID : Subsystem
  ReferenceFrame : sm_lib/Frames and Transforms/Reference Frame
  F : PMIOPort  Side=Left
  F1 : PMIOPort  Port=2  Side=Right
  connections:
  Arbre_Poignet_1_RIGID/LConn3 -- Assemblage_Parfait_1/LConn1
  Arbre_Poignet_1_RIGID/LConn2 -- Part_2_1_RIGID/LConn2
  Arbre_Poignet_1_RIGID/LConn1 -- Goupille_1_RIGID/LConn1
  Part_2_1_RIGID/LConn1 -- F/RConn1
  F1/RConn1 -- Assemblage_Parfait_1/RConn1

== system Moteurs_PLA/Robot/Base ==
  Base_1_RIGID : Subsystem
  Couvercle_1_RIGID : Subsystem
  Joints_1_RIGID : Subsystem
  F : PMIOPort  Side=Right
  F2 : PMIOPort  Port=2  Side=Left
  connections:
  Base_1_RIGID/LConn1 -- Joints_1_RIGID/LConn1
  Base_1_RIGID/LConn3 -- Couvercle_1_RIGID/LConn1
  Joints_1_RIGID/RConn1 -- F/RConn1
  F2/RConn1 -- Base_1_RIGID/LConn2

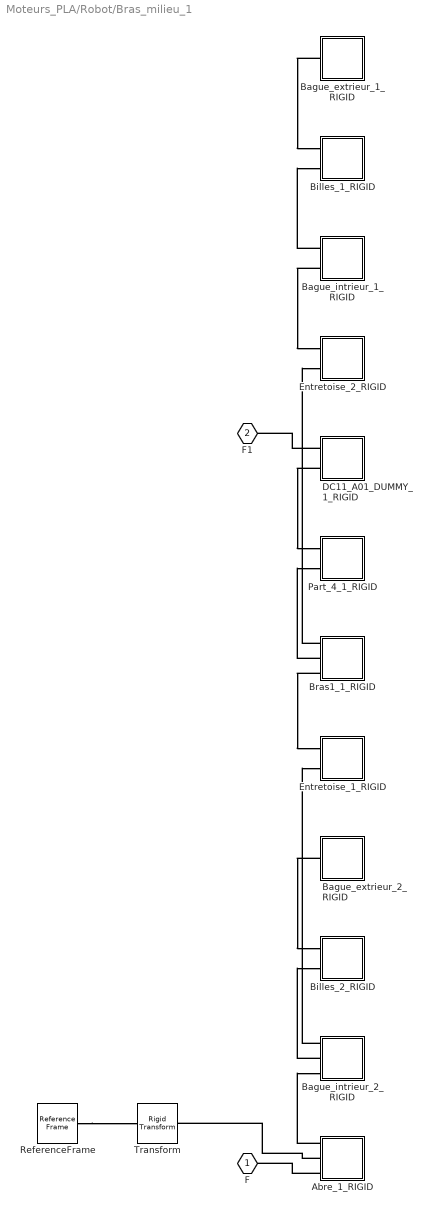
== system Moteurs_PLA/Robot/Bras_milieu_1 ==
  Abre_1_RIGID : Subsystem
  Bague_extrieur_1_RIGID : Subsystem
  Bague_extrieur_2_RIGID : Subsystem
  Bague_intrieur_1_RIGID : Subsystem
  Bague_intrieur_2_RIGID : Subsystem
  Billes_1_RIGID : Subsystem
  Billes_2_RIGID : Subsystem
  Bras1_1_RIGID : Subsystem
  DC11_A01_DUMMY_1_RIGID : Subsystem
  Entretoise_1_RIGID : Subsystem
  Entretoise_2_RIGID : Subsystem
  Part_4_1_RIGID : Subsystem
  ReferenceFrame : sm_lib/Frames and Transforms/Reference Frame
  Transform : sm_lib/Frames and Transforms/Rigid Transform  TranslationMethod=Cartesian  TranslationStandardOffset=0  TranslationLengthUnit=m  TranslationStandardAxis=+Z  TranslationCartesianOffset=smiData.RigidTransform(95).translation  TranslationROffset=0  TranslationROffsetUnits=m  TranslationZOffset=0  TranslationZOffsetUnits=m  TranslationThetaOffset=0  TranslationThetaOffsetUnits=deg  RotationMethod=ArbitraryAxis  RotationAngleUnits=rad  RotationStandardAxis=+Z  RotationAngle=smiData.RigidTransform(95).angle  RotationArbitraryAxis=smiData.RigidTransform(95).axis  FollAlignAxisA=+X  BaseAlignAxisA=+Y  FollAlignAxisB=+Y  BaseAlignAxisB=+Z  RotationSequenceAxes=FollowerAxes  RotationSequence=XYX  RotationSequenceAngles=[0 0 0]  RotationSequenceAnglesUnits=deg  RotationMatrix=[1 0 0; 0 1 0; 0 0 1]
  F : PMIOPort  Side=Left
  F1 : PMIOPort  Port=2  Side=Right
  connections:
  Abre_1_RIGID/LConn1 -- Bague_intrieur_2_RIGID/LConn3
  Bras1_1_RIGID/LConn2 -- Part_4_1_RIGID/LConn2
  Bague_intrieur_1_RIGID/LConn2 -- Entretoise_2_RIGID/LConn1
  Abre_1_RIGID/LConn3 -- F/RConn1
  DC11_A01_DUMMY_1_RIGID/LConn1 -- F1/RConn1
  Abre_1_RIGID/LConn2 -- Transform/RConn1
  ReferenceFrame/RConn1 -- Transform/LConn1
  DC11_A01_DUMMY_1_RIGID/LConn2 -- Part_4_1_RIGID/LConn1
  Bague_extrieur_2_RIGID/LConn1 -- Billes_2_RIGID/LConn1
  Bague_intrieur_2_RIGID/LConn2 -- Billes_2_RIGID/LConn2
  Bras1_1_RIGID/LConn3 -- Entretoise_1_RIGID/LConn1
  Bras1_1_RIGID/LConn1 -- Entretoise_2_RIGID/LConn2
  Bague_extrieur_1_RIGID/LConn1 -- Billes_1_RIGID/LConn1
  Bague_intrieur_1_RIGID/LConn1 -- Billes_1_RIGID/LConn2
  Bague_intrieur_2_RIGID/LConn1 -- Entretoise_1_RIGID/LConn2

== system Moteurs_PLA/Robot/Moteur_bassin_1 ==
  Bras0_1_RIGID : Subsystem
  Bras0_2_RIGID : Subsystem
  Fixation_moteur_1_RIGID : Subsystem
  Moteur_1_RIGID : Subsystem
  Mt_1_RIGID : Subsystem
  ReferenceFrame : sm_lib/Frames and Transforms/Reference Frame
  F1 : PMIOPort  Side=Left
  F : PMIOPort  Port=2  Side=Right
  connections:
  Bras0_1_RIGID/LConn2 -- Mt_1_RIGID/LConn1
  Bras0_1_RIGID/LConn1 -- Fixation_moteur_1_RIGID/LConn2
  Bras0_2_RIGID/LConn1 -- Mt_1_RIGID/LConn3
  Fixation_moteur_1_RIGID/LConn1 -- Moteur_1_RIGID/LConn2
  Moteur_1_RIGID/LConn1 -- F/RConn1
  Mt_1_RIGID/LConn2 -- F1/RConn1

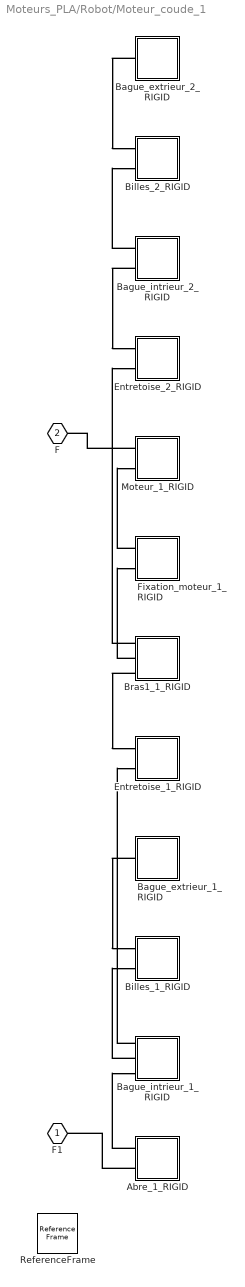
== system Moteurs_PLA/Robot/Moteur_coude_1 ==
  Abre_1_RIGID : Subsystem
  Bague_extrieur_1_RIGID : Subsystem
  Bague_extrieur_2_RIGID : Subsystem
  Bague_intrieur_1_RIGID : Subsystem
  Bague_intrieur_2_RIGID : Subsystem
  Billes_1_RIGID : Subsystem
  Billes_2_RIGID : Subsystem
  Bras1_1_RIGID : Subsystem
  Entretoise_1_RIGID : Subsystem
  Entretoise_2_RIGID : Subsystem
  Fixation_moteur_1_RIGID : Subsystem
  Moteur_1_RIGID : Subsystem
  ReferenceFrame : sm_lib/Frames and Transforms/Reference Frame
  F1 : PMIOPort  Side=Left
  F : PMIOPort  Port=2  Side=Right
  connections:
  Bras1_1_RIGID/LConn1 -- Entretoise_2_RIGID/LConn2
  Bras1_1_RIGID/LConn3 -- Entretoise_1_RIGID/LConn1
  Bague_intrieur_2_RIGID/LConn1 -- Billes_2_RIGID/LConn2
  Moteur_1_RIGID/LConn1 -- F/RConn1
  Abre_1_RIGID/LConn2 -- F1/RConn1
  Bras1_1_RIGID/LConn2 -- Fixation_moteur_1_RIGID/LConn2
  Fixation_moteur_1_RIGID/LConn1 -- Moteur_1_RIGID/LConn2
  Bague_extrieur_1_RIGID/LConn1 -- Billes_1_RIGID/LConn1
  Bague_intrieur_1_RIGID/LConn2 -- Billes_1_RIGID/LConn2
  Abre_1_RIGID/LConn1 -- Bague_intrieur_1_RIGID/LConn3
  Bague_extrieur_2_RIGID/LConn1 -- Billes_2_RIGID/LConn1
  Bague_intrieur_2_RIGID/LConn2 -- Entretoise_2_RIGID/LConn1
  Bague_intrieur_1_RIGID/LConn1 -- Entretoise_1_RIGID/LConn2

== system Moteurs_PLA/Robot/Moteur_poignet_1 ==
  Arbre_Poignet_1_RIGID : Subsystem
  Assemblage_Parfait_1 : Subsystem
  Goupille_1_RIGID : Subsystem
  Part_2_1_RIGID : Subsystem
  ReferenceFrame : sm_lib/Frames and Transforms/Reference Frame
  F : PMIOPort  Side=Left
  F1 : PMIOPort  Port=2  Side=Right
  connections:
  Arbre_Poignet_1_RIGID/LConn3 -- Assemblage_Parfait_1/LConn1
  Arbre_Poignet_1_RIGID/LConn2 -- Part_2_1_RIGID/LConn2
  Arbre_Poignet_1_RIGID/LConn1 -- Goupille_1_RIGID/LConn1
  Part_2_1_RIGID/LConn1 -- F/RConn1
  F1/RConn1 -- Assemblage_Parfait_1/RConn1

== system Moteurs_PLA/Bras/Base/Base_1_RIGID ==
  ReferenceFrame : sm_lib/Frames and Transforms/Reference Frame
  Solid : sm_lib/Body Elements/File Solid  ExtGeomFileName=Base.step  UnitType=FromFile  ExtGeomFileUnits=m  StepReaderType=HEX  ExportConvexHullGeometry=off  InertiaType=Custom  Mass=smiData.Solid(1).mass  MassUnits=kg  CenterOfMass=smiData.Solid(1).CoM  CenterOfMassUnits=m  MomentsOfInertia=smiData.Solid(1).MoI  MomentsOfInertiaUnits=kg*m^2  ProductsOfInertia=smiData.Solid(1).PoI  ProductsOfInertiaUnits=kg*m^2  BasedOnType=DensityFromFile  Density=1000  DensityUnits=kg/m^3  DoExposeReferenceFrame=on  SerializedFrames=<Frames/>  GraphicType=FromGeometry  MarkerShape=Sphere  MarkerSize=10  GraphicVisPropType=SimpleVisualProperties  GraphicDiffuseColor=smiData.Solid(1).color  GraphicSpecularColor=[0.5 0.5 0.5 1.0]  GraphicAmbientColor=[0.15 0.15 0.15 1.0]  GraphicEmissiveColor=[0.0 0.0 0.0 1.0]  GraphicShininess=75  GraphicOpacity=smiData.Solid(1).opacity
  Transform : sm_lib/Frames and Transforms/Rigid Transform  TranslationMethod=Cartesian  TranslationStandardOffset=0  TranslationLengthUnit=m  TranslationStandardAxis=+Z  TranslationCartesianOffset=smiData.RigidTransform(85).translation  TranslationROffset=0  TranslationROffsetUnits=m  TranslationZOffset=0  TranslationZOffsetUnits=m  TranslationThetaOffset=0  TranslationThetaOffsetUnits=deg  RotationMethod=ArbitraryAxis  RotationAngleUnits=rad  RotationStandardAxis=+Z  RotationAngle=smiData.RigidTransform(85).angle  RotationArbitraryAxis=smiData.RigidTransform(85).axis  FollAlignAxisA=+X  BaseAlignAxisA=+Y  FollAlignAxisB=+Y  BaseAlignAxisB=+Z  RotationSequenceAxes=FollowerAxes  RotationSequence=XYX  RotationSequenceAngles=[0 0 0]  RotationSequenceAnglesUnits=deg  RotationMatrix=[1 0 0; 0 1 0; 0 0 1]
  Transform1 : sm_lib/Frames and Transforms/Rigid Transform  TranslationMethod=Cartesian  TranslationStandardOffset=0  TranslationLengthUnit=m  TranslationStandardAxis=+Z  TranslationCartesianOffset=smiData.RigidTransform(91).translation  TranslationROffset=0  TranslationROffsetUnits=m  TranslationZOffset=0  TranslationZOffsetUnits=m  TranslationThetaOffset=0  TranslationThetaOffsetUnits=deg  RotationMethod=ArbitraryAxis  RotationAngleUnits=rad  RotationStandardAxis=+Z  RotationAngle=smiData.RigidTransform(91).angle  RotationArbitraryAxis=smiData.RigidTransform(91).axis  FollAlignAxisA=+X  BaseAlignAxisA=+Y  FollAlignAxisB=+Y  BaseAlignAxisB=+Z  RotationSequenceAxes=FollowerAxes  RotationSequence=XYX  RotationSequenceAngles=[0 0 0]  RotationSequenceAnglesUnits=deg  RotationMatrix=[1 0 0; 0 1 0; 0 0 1]
  F1 : PMIOPort  Side=Left
  F2 : PMIOPort  Port=2  Side=Left
  F : PMIOPort  Port=3  Side=Left
  connections:
  ReferenceFrame/RConn1 -- Solid/RConn1 -- Transform/LConn1 -- Transform1/LConn1 -- F2/RConn1
  Transform/RConn1 -- F/RConn1
  Transform1/RConn1 -- F1/RConn1

== system Moteurs_PLA/Bras/Base/Couvercle_1_RIGID ==
  ReferenceFrame : sm_lib/Frames and Transforms/Reference Frame
  Solid : sm_lib/Body Elements/File Solid  ExtGeomFileName=Couvercle.step  UnitType=FromFile  ExtGeomFileUnits=m  StepReaderType=HEX  ExportConvexHullGeometry=off  InertiaType=Custom  Mass=smiData.Solid(7).mass  MassUnits=kg  CenterOfMass=smiData.Solid(7).CoM  CenterOfMassUnits=m  MomentsOfInertia=smiData.Solid(7).MoI  MomentsOfInertiaUnits=kg*m^2  ProductsOfInertia=smiData.Solid(7).PoI  ProductsOfInertiaUnits=kg*m^2  BasedOnType=DensityFromFile  Density=1000  DensityUnits=kg/m^3  DoExposeReferenceFrame=on  SerializedFrames=<Frames/>  GraphicType=FromGeometry  MarkerShape=Sphere  MarkerSize=10  GraphicVisPropType=SimpleVisualProperties  GraphicDiffuseColor=smiData.Solid(7).color  GraphicSpecularColor=[0.5 0.5 0.5 1.0]  GraphicAmbientColor=[0.15 0.15 0.15 1.0]  GraphicEmissiveColor=[0.0 0.0 0.0 1.0]  GraphicShininess=75  GraphicOpacity=smiData.Solid(7).opacity
  Transform : sm_lib/Frames and Transforms/Rigid Transform  TranslationMethod=Cartesian  TranslationStandardOffset=0  TranslationLengthUnit=m  TranslationStandardAxis=+Z  TranslationCartesianOffset=smiData.RigidTransform(86).translation  TranslationROffset=0  TranslationROffsetUnits=m  TranslationZOffset=0  TranslationZOffsetUnits=m  TranslationThetaOffset=0  TranslationThetaOffsetUnits=deg  RotationMethod=ArbitraryAxis  RotationAngleUnits=rad  RotationStandardAxis=+Z  RotationAngle=smiData.RigidTransform(86).angle  RotationArbitraryAxis=smiData.RigidTransform(86).axis  FollAlignAxisA=+X  BaseAlignAxisA=+Y  FollAlignAxisB=+Y  BaseAlignAxisB=+Z  RotationSequenceAxes=FollowerAxes  RotationSequence=XYX  RotationSequenceAngles=[0 0 0]  RotationSequenceAnglesUnits=deg  RotationMatrix=[1 0 0; 0 1 0; 0 0 1]
  F : PMIOPort  Side=Left
  connections:
  ReferenceFrame/RConn1 -- Solid/RConn1 -- Transform/LConn1
  Transform/RConn1 -- F/RConn1
